simulink model "c_KCL"  (R2024b)
settings: Solver=ode15s  StartTime=0.0  StopTime=Tsim  RelTol=1e-3
model workspace (MAT data in the model file):
  C_1 = 1
  C_2 = 1
  C_3 = 1
  L_1 = 1
  L_2 = 1
  L_3 = 1
  Len_1 = 0.001
  Len_2 = 0.001
  Len_3 = 0.001
  R_1 = 30
  R_2 = 20
  R_3 = 500
  R_c_1 = 500
  R_c_2 = 500
  R_c_3 = 500
  Tsim = 0.0001
  Tstep = 5e-05
  dtMax = 1e-06
libraries: nesl_utility x13, fl_lib x9, ODEsim x3
settings Model: Creator=cao2851  LastModifiedBy=cao2851
settings DataIOCC: ExternalInput=ds{1}  LoadExternalInput=on

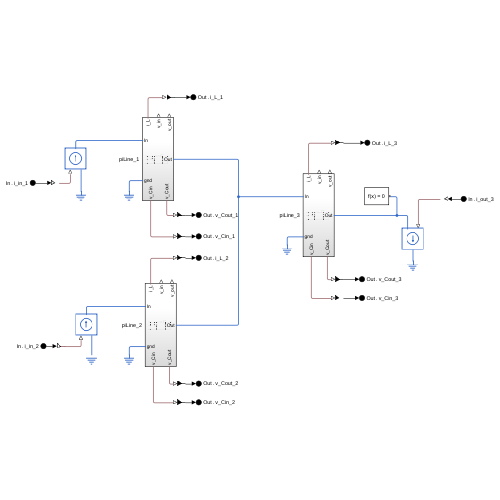
[thumbnail: Simulink's stored preview of the top-level diagram]
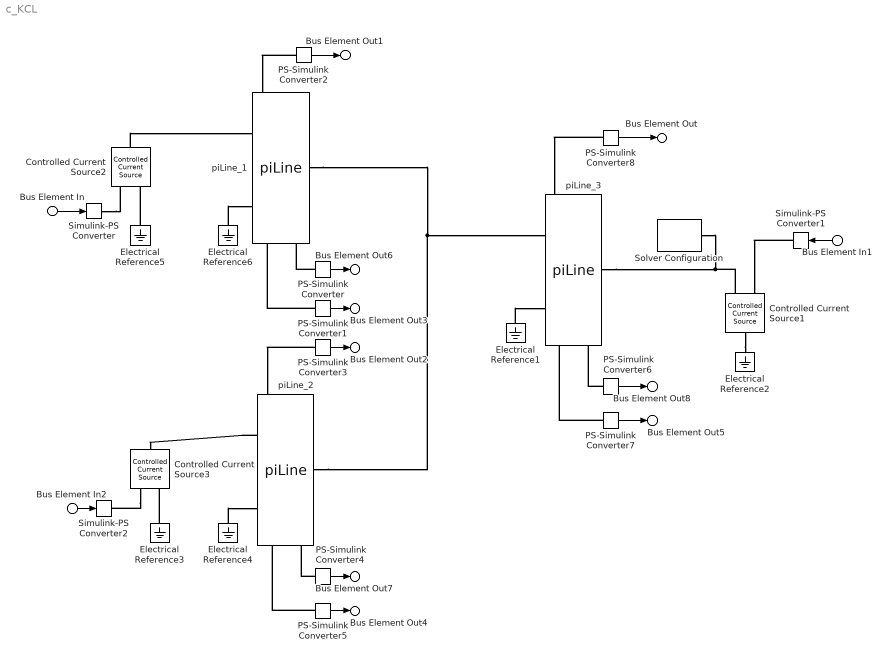
== system c_KCL ==
  Bus Element In : Inport  PortName=In  Element=i_in_1
  Bus Element In1 : Inport  PortName=In  Element=i_out_3
  Bus Element In2 : Inport  PortName=In  Element=i_in_2
  Controlled Current Source1 : fl_lib/Electrical/Electrical Sources/Controlled Current Source
  Controlled Current Source2 : fl_lib/Electrical/Electrical Sources/Controlled Current Source
  Controlled Current Source3 : fl_lib/Electrical/Electrical Sources/Controlled Current Source
  Electrical Reference{1..6} (6 alike) : fl_lib/Electrical/Electrical Elements/Electrical Reference
  PS-Simulink Converter{,1..8} (9 alike) : nesl_utility/PS-Simulink Converter  PhysicalDomain=network_engine_domain  SubClassName=ps_output  LeftPortType=input  RightPortType=output  PseudoPeriodic=off  Frequencies=[]  VectorFormat=inherit  Unit=inherit  AffineConversion=off
  Simulink-PS Converter : nesl_utility/Simulink-PS Converter  PhysicalDomain=network_engine_domain  SubClassName=ps_input  LeftPortType=input  RightPortType=output  PseudoPeriodic=off  Frequencies=[]  NoiseDistribution=none  NoiseParameters=[]  Unit=1  AffineConversion=off  FilteringAndDerivatives=zero  SimscapeFilterOrder=1  InputFilterTimeConstant=0.001  UdotUserProvided=0
  Simulink-PS Converter1 : nesl_utility/Simulink-PS Converter  PhysicalDomain=network_engine_domain  SubClassName=ps_input  LeftPortType=input  RightPortType=output  PseudoPeriodic=off  Frequencies=[]  NoiseDistribution=none  NoiseParameters=[]  Unit=1  AffineConversion=off  FilteringAndDerivatives=zero  SimscapeFilterOrder=1  InputFilterTimeConstant=0.001  UdotUserProvided=0
  Simulink-PS Converter2 : nesl_utility/Simulink-PS Converter  PhysicalDomain=network_engine_domain  SubClassName=ps_input  LeftPortType=input  RightPortType=output  PseudoPeriodic=off  Frequencies=[]  NoiseDistribution=none  NoiseParameters=[]  Unit=1  AffineConversion=off  FilteringAndDerivatives=zero  SimscapeFilterOrder=1  InputFilterTimeConstant=0.001  UdotUserProvided=0
  Solver Configuration : nesl_utility/Solver Configuration  PhysicalDomain=network_engine_domain  SubClassName=solver  LeftPortType=input  RightPortType=generic  Tones=[]  Harmonics=[]  SimulateNoise=off  Profile=off  UseLocalSampling=off  EnableSwitchedLinearOptims=on  FrequencyDomain=off  UseCCode=off  RelTol=0.001  AbsTol=0.001  MinStep=1e-09  ToWorkspace=off  RevertToSquareIcSolve=off  NumHomotopyIterations=100  PhasorMode=off  PhasorModeNumHarmonics=1  ConsistencySolver=NEWTON_XTOL_AFTER_FTOL  IndexReductionMethod=DerivativeReplacement  DoDC=off  ResidualTolerance=1e-09  ConsistencyTolSource=GLOBAL  ConsistencyAbsTol=0.001  ConsistencyRelTol=0.001  ConsistencyTolFactor=1e-6  UseLocalSolver=off  LocalSolverChoice=NE_BACKWARD_EULER_ADVANCER  ResolveIndetEquations=on  FunctionEvalNumThread=1  LocalSolverSampleTime=0.001  DoFixedCost=off  MaxNonlinIter=3  MaxModeIter=2  ComputeImpulses=off  ImpulseIterations=2  LinearAlgebra=auto  LinearAlgebraNumThread=0  EquationFormulation=NE_TIME_EF  DelaysMemoryBudget=1024  AutomaticFiltering=on  FilteringTimeConstant=0.001  PartitionStorageMethod=AS_NEEDED  PartitionMemoryBudget=1024  PartitionMethod=ROBUST  MultibodyUseLocalSolver=off  MultibodyLocalSolverChoice=ODE1  MultibodyLocalSolverSampleTime=0.001
  piLine_1 : ODEsim/piLine  SystemSampleTime=-1  VariantActivationTime=update diagram  AllowFlexibleInterface=on  Latency=0  AutoFrameSizeCalculation=off
      link override Cline1: c=C_1 / 2 * Len_1
      link override Cline1_r: R=R_c_1
      link override Cline2: c=C_1 / 2 * Len_1
      link override Cline2_r: R=R_c_1
      link override Lline: l=L_1 * Len_1
      link override Rline: R=R_1 * Len_1
      settings: PortSchema="{\"entries\":[{\"content\":{\"sides\":[{\"content\":{\"connectorIds\":[\"LConn1\",\"LConn2\"]},\"type\":\"ConnectorPlacement.EquallySpacedRectSide\",\"uuid\":\"2f581a64-5488-4115-8fb4-4c7dc7f7cc02\"},{\"content\":{\"connectorIds\":[\"RConn1\"],\"side\":\"RIGHT\"},\"type\":\"ConnectorPlacement.EquallySpacedRectSide\",\"uuid\":\"41fc3ed1-c08d-4cec-81c4-9e5ea37f4b50\"},{\"content\":{\"connectorIds\":[\"LConn3\",\"LConn4\",\"LConn5\"],\"side\":\"TOP\"},\"type\":\"ConnectorPlacement.EquallySpacedRectSide\",\"uuid\":\"f632da0e-7244-44f2-8232-d25344579225\"},{\"content\":{\"connectorIds\":[\"RConn2\",\"RConn3\"],\"side\":\"BOTTOM\"},\"type\":\"ConnectorPlacement.EquallySpacedRectSide\",\"uuid\":\"4895b748-0fce-4270-baa5-001cc2b4bab4\"}]},\"type\":\"ConnectorPlacement.EquallySpacedConnector\",\"uuid\":\"08f1579d-6e1b-4490-ba48-7710ed18f2cd\"}],\"packageUris\":[\"http://schema.mathworks.com/mf0/Connector/R2020b\"],\"version\":\"1.0\"}"
  piLine_2 : ODEsim/piLine  SystemSampleTime=-1  VariantActivationTime=update diagram  AllowFlexibleInterface=on  Latency=0  AutoFrameSizeCalculation=off
      link override Cline1: c=C_2 / 2 * Len_2
      link override Cline1_r: R=R_c_2
      link override Cline2: c=C_2 / 2 * Len_2
      link override Cline2_r: R=R_c_2
      link override Lline: l=L_2 * Len_2
      link override Rline: R=R_2 * Len_2
      settings: PortSchema="{\"entries\":[{\"content\":{\"sides\":[{\"content\":{\"connectorIds\":[\"LConn1\",\"LConn2\"]},\"type\":\"ConnectorPlacement.EquallySpacedRectSide\",\"uuid\":\"2f581a64-5488-4115-8fb4-4c7dc7f7cc02\"},{\"content\":{\"connectorIds\":[\"RConn1\"],\"side\":\"RIGHT\"},\"type\":\"ConnectorPlacement.EquallySpacedRectSide\",\"uuid\":\"41fc3ed1-c08d-4cec-81c4-9e5ea37f4b50\"},{\"content\":{\"connectorIds\":[\"LConn3\",\"LConn4\",\"LConn5\"],\"side\":\"TOP\"},\"type\":\"ConnectorPlacement.EquallySpacedRectSide\",\"uuid\":\"f632da0e-7244-44f2-8232-d25344579225\"},{\"content\":{\"connectorIds\":[\"RConn2\",\"RConn3\"],\"side\":\"BOTTOM\"},\"type\":\"ConnectorPlacement.EquallySpacedRectSide\",\"uuid\":\"4895b748-0fce-4270-baa5-001cc2b4bab4\"}]},\"type\":\"ConnectorPlacement.EquallySpacedConnector\",\"uuid\":\"08f1579d-6e1b-4490-ba48-7710ed18f2cd\"}],\"packageUris\":[\"http://schema.mathworks.com/mf0/Connector/R2020b\"],\"version\":\"1.0\"}"
  piLine_3 : ODEsim/piLine  SystemSampleTime=-1  VariantActivationTime=update diagram  AllowFlexibleInterface=on  Latency=0  AutoFrameSizeCalculation=off
      link override Cline1: c=C_3 / 2 * Len_3
      link override Cline1_r: R=R_c_3
      link override Cline2: c=C_3 / 2 * Len_3
      link override Cline2_r: R=R_c_3
      link override Lline: l=L_3 * Len_3
      link override Rline: R=R_3 * Len_3
      settings: PortSchema="{\"entries\":[{\"content\":{\"sides\":[{\"content\":{\"connectorIds\":[\"LConn1\",\"LConn2\"]},\"type\":\"ConnectorPlacement.EquallySpacedRectSide\",\"uuid\":\"2f581a64-5488-4115-8fb4-4c7dc7f7cc02\"},{\"content\":{\"connectorIds\":[\"RConn1\"],\"side\":\"RIGHT\"},\"type\":\"ConnectorPlacement.EquallySpacedRectSide\",\"uuid\":\"41fc3ed1-c08d-4cec-81c4-9e5ea37f4b50\"},{\"content\":{\"connectorIds\":[\"LConn3\",\"LConn4\",\"LConn5\"],\"side\":\"TOP\"},\"type\":\"ConnectorPlacement.EquallySpacedRectSide\",\"uuid\":\"f632da0e-7244-44f2-8232-d25344579225\"},{\"content\":{\"connectorIds\":[\"RConn2\",\"RConn3\"],\"side\":\"BOTTOM\"},\"type\":\"ConnectorPlacement.EquallySpacedRectSide\",\"uuid\":\"4895b748-0fce-4270-baa5-001cc2b4bab4\"}]},\"type\":\"ConnectorPlacement.EquallySpacedConnector\",\"uuid\":\"08f1579d-6e1b-4490-ba48-7710ed18f2cd\"}],\"packageUris\":[\"http://schema.mathworks.com/mf0/Connector/R2020b\"],\"version\":\"1.0\"}"
  Bus Element Out : Outport  PortName=Out  Element=i_L_3
  Bus Element Out1 : Outport  PortName=Out  Element=i_L_1
  Bus Element Out2 : Outport  PortName=Out  Element=i_L_2
  Bus Element Out3 : Outport  PortName=Out  Element=v_Cin_1
  Bus Element Out4 : Outport  PortName=Out  Element=v_Cin_2
  Bus Element Out5 : Outport  PortName=Out  Element=v_Cin_3
  Bus Element Out6 : Outport  PortName=Out  Element=v_Cout_1
  Bus Element Out7 : Outport  PortName=Out  Element=v_Cout_2
  Bus Element Out8 : Outport  PortName=Out  Element=v_Cout_3
  wires:
  Bus Element In/1 -> Simulink-PS Converter/1
  Bus Element In1/1 -> Simulink-PS Converter1/1
  Bus Element In2/1 -> Simulink-PS Converter2/1
  PS-Simulink Converter8/1 -> Bus Element Out/1
  PS-Simulink Converter2/1 -> Bus Element Out1/1
  PS-Simulink Converter3/1 -> Bus Element Out2/1
  PS-Simulink Converter1/1 -> Bus Element Out3/1
  PS-Simulink Converter5/1 -> Bus Element Out4/1
  PS-Simulink Converter7/1 -> Bus Element Out5/1
  PS-Simulink Converter/1 -> Bus Element Out6/1
  PS-Simulink Converter4/1 -> Bus Element Out7/1
  PS-Simulink Converter6/1 -> Bus Element Out8/1
  connections:
  Controlled Current Source1/LConn1 -- Electrical Reference2/LConn1
  Simulink-PS Converter1/RConn1 -- Controlled Current Source1/RConn1
  Solver Configuration/RConn1 -- Controlled Current Source1/RConn2 -- piLine_3/RConn1
  Simulink-PS Converter/RConn1 -- Controlled Current Source2/RConn1
  Controlled Current Source3/RConn1 -- Simulink-PS Converter2/RConn1
  piLine_2/LConn1 -- Controlled Current Source3/LConn1
  Electrical Reference3/LConn1 -- Controlled Current Source3/RConn2
  Electrical Reference4/LConn1 -- piLine_2/LConn2
  Electrical Reference1/LConn1 -- piLine_3/LConn2
  piLine_1/RConn1 -- piLine_2/RConn1 -- piLine_3/LConn1
  Controlled Current Source2/LConn1 -- piLine_1/LConn1
  Electrical Reference5/LConn1 -- Controlled Current Source2/RConn2
  Electrical Reference6/LConn1 -- piLine_1/LConn2
  PS-Simulink Converter/LConn1 -- piLine_1/RConn3
  PS-Simulink Converter1/LConn1 -- piLine_1/RConn2
  PS-Simulink Converter2/LConn1 -- piLine_1/LConn3
  PS-Simulink Converter3/LConn1 -- piLine_2/LConn3
  PS-Simulink Converter4/LConn1 -- piLine_2/RConn3
  PS-Simulink Converter5/LConn1 -- piLine_2/RConn2
  PS-Simulink Converter6/LConn1 -- piLine_3/RConn3
  PS-Simulink Converter7/LConn1 -- piLine_3/RConn2
  PS-Simulink Converter8/LConn1 -- piLine_3/LConn3
